simulink model "thermal_model_pwm"  (R2024a)
settings: Solver=VariableStepAuto  StartTime=0.0  StopTime=10000  RelTol=1e-3
settings Model: Creator=DuRuofu  LastModifiedBy=DuRuofu

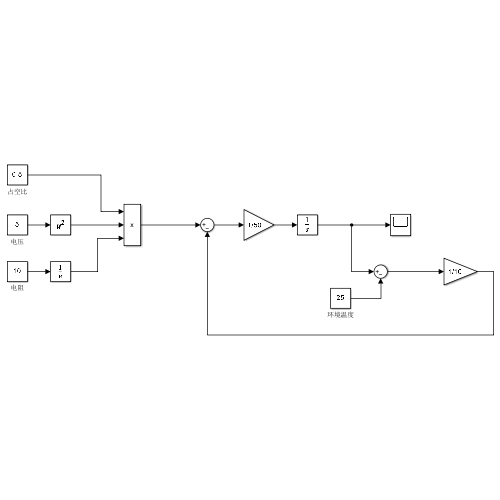
[thumbnail: Simulink's stored preview of the top-level diagram]
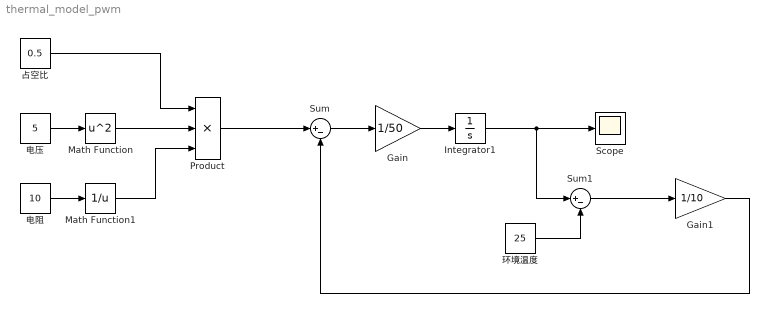
== system thermal_model_pwm ==
  Gain : Gain  Gain=1/50
  Gain1 : Gain  Gain=1/10
  Integrator1 : Integrator  InitialCondition=25
  Math Function : Math  Operator=square
  Math Function1 : Math  Operator=reciprocal
  Product : Product  Inputs=3
  Scope : Scope
  Sum : Sum  Inputs=|+-
  Sum1 : Sum  Inputs=|+-
  占空比 : Constant  Value=0.5
  环境温度 : Constant  Value=25
  电压 : Constant  Value=5
  电阻 : Constant  Value=10
  wires:
  电压/1 -> Math Function/1
  占空比/1 -> Product/1
  Math Function/1 -> Product/2
  Product/1 -> Sum/1
  电阻/1 -> Math Function1/1
  Math Function1/1 -> Product/3
  Sum/1 -> Gain/1
  Gain/1 -> Integrator1/1
  Integrator1/1 -> Sum1/1, Scope/1
  环境温度/1 -> Sum1/2
  Sum1/1 -> Gain1/1
  Gain1/1 -> Sum/2
